simulink model "untitle"  (R2023a)
settings: Solver=VariableStepAuto  StartTime=0.0  StopTime=10.0  RelTol=1e-3
libraries: spsWindTurbineLib x1
settings Model: Creator=satyajeet tripathy  LastModifiedBy=satyajeet tripathy

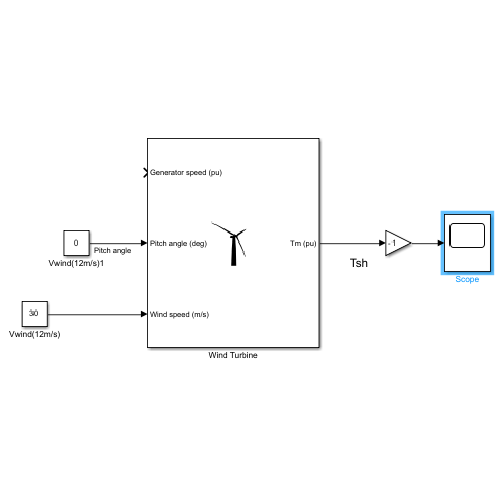
[thumbnail: Simulink's stored preview of the top-level diagram]
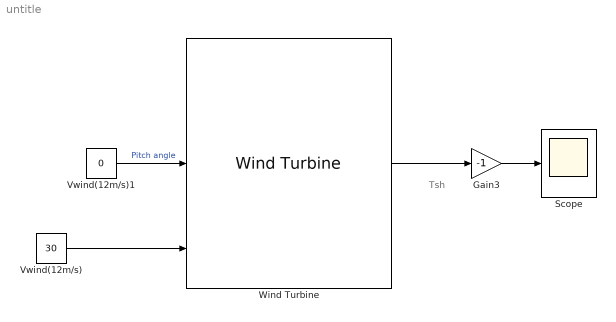
== system untitle ==
  note: Tsh
  Gain3 : Gain  Gain=-1
  Scope : Scope
  Vwind(12m/s) : Constant  Value=30
  Vwind(12m/s)1 : Constant  Value=0
  Wind Turbine : spsWindTurbineLib/Wind Turbine  Pnom=8.5e3  Pelec_base=8.5e3/0.9  wind_base=20  P_wind_base=0.8  speed_nom=1  pitch_angle=0  c1_c6="[0.51763          116          0.4            5           21     0.006795]"  cp_nom=0.48  lambda_nom=8.1
  wires:
  Wind Turbine/1 -> Gain3/1
  Vwind(12m/s)/1 -> Wind Turbine/3
  Vwind(12m/s)1/1 -> Wind Turbine/2  "Pitch angle"
  Gain3/1 -> Scope/1
